simulink model "GlobalMPC"  (R2022b)
settings: Solver=FixedStepAuto  StartTime=0.0  StopTime=3600  FixedStep=3600  RelTol=1e-3
values from neighbouring files (symbols this model uses):
  c = scaled_standard_constants    [Run_simulation.m]
settings Model: Creator=is123  LastModifiedBy=is123
settings OptimizationCC: ReuseModelBlockBuffer=on

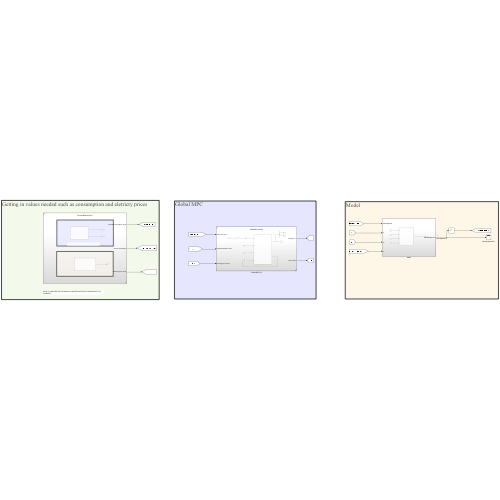
[thumbnail: Simulink's stored preview of the top-level diagram]
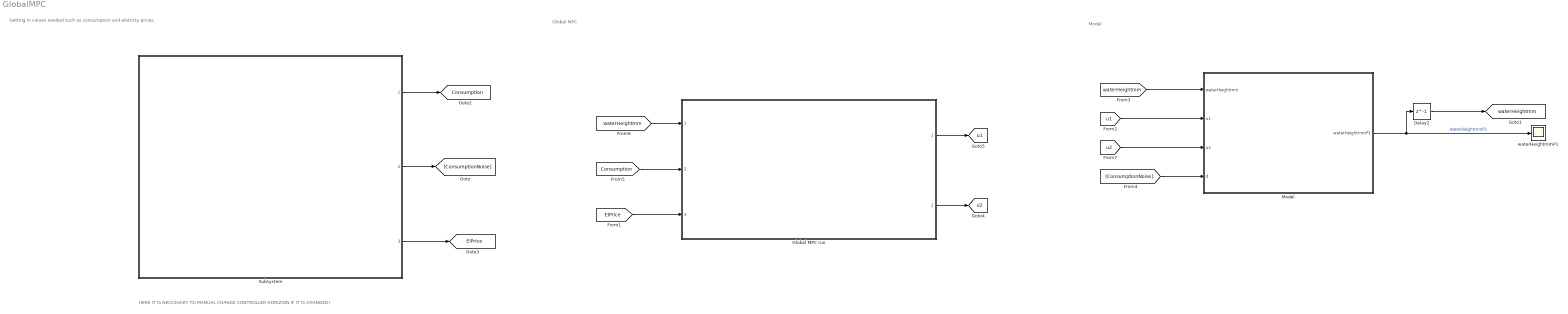
== system GlobalMPC ==
  note: Getting in values needed such as consumption and eletricty prices
  note: Global MPC
  note: Model
  note: HERE IT IS NECCESARY TO MANUAL CHANGE CONTROLLER HORIZION IF IT IS CHANGED!
  Delay2 : Delay  DelayLength=1  InitialCondition=c.V/c.At*1e3
  Global MPC run : Subsystem  ReferencedSubsystem=GlobalMPController
  Model : Subsystem
  Subsystem : Subsystem  ReferencedSubsystem=DemandEletricityPrice
  waterHeightmmP1 : Scope
  tag scope: Consumption=global, ElPrice=global, u1=global, u2=global, waterHeightmm=global
  wires:
  Model/1(waterHeightmmP1) -> Delay2/1, waterHeightmmP1/1  "waterHeightmmP1"
  [waterHeightmm] -> Model/1(waterHeightmm)
  Delay2/1 -> [waterHeightmm]
  [u1] -> Model/2(u1)
  [ConsumptionNoise] -> Model/4(d)
  Global MPC run/1 -> [u1]
  Subsystem/2 -> [ConsumptionNoise]
  Subsystem/1 -> [Consumption]
  Subsystem/3 -> [ElPrice]
  [waterHeightmm] -> Global MPC run/1
  [Consumption] -> Global MPC run/2
  [ElPrice] -> Global MPC run/3
  Global MPC run/2 -> [u2]
  [u2] -> Model/3(u2)

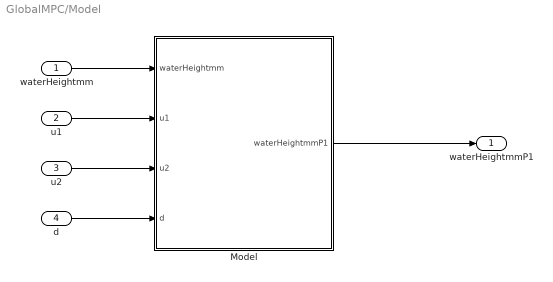
== system GlobalMPC/Model ==
  waterHeightmm : Inport
  u1 : Inport  Port=2
  u2 : Inport  Port=3
  d : Inport  Port=4
  Model : MATLAB Function  TreatAsAtomicUnit=on  SystemSampleTime=3600/c.AccTime
  waterHeightmmP1 : Outport
  wires:
  Model/1(waterHeightmmP1) -> waterHeightmmP1/1
  waterHeightmm/1 -> Model/1(waterHeightmm)
  u1/1 -> Model/2(u1)
  d/1 -> Model/4(d)
  u2/1 -> Model/3(u2)

== matlab function GlobalMPC/Model/Model ==
  data: waterHeightmm input; u1 input; u2 input; waterHeightmmP1 output; d input
function waterHeightmmP1 = model(waterHeightmm,u1,u2,d)
%Caling the model function
%Setting the output to zero becuase it is needed
c=standardConstants;

waterHeightmmP1=zeros(1,1); 
u=[u1;u2];
%calling the model function to get the next volumen
V=waterHeightmm/1e3*c.At;

Vp1=Model(V,u,d);

waterHeightmmP1=Vp1/c.At*1e3; 

end
